simulink model "tp14"  (R2024b)
settings: Solver=ode23t  StartTime=0.0  StopTime=0.2  FixedStep=0.2  RelTol=1e-4  AbsTol=1e-6  EnableMultiTasking=on
undefined symbols (not defined in the file or in its folder): D1, Delta
libraries: spsThreePhaseVIMeasurementLib x28, spsThreePhaseSeriesRLCBranchLib x20, simulink x14, eePMU x14, spsThreePhaseSeriesRLCLoadLib x11, spsThreePhaseSourceLib x5, spsThreePhaseTransformerTwoWindingsLib x5, spspowerguiLib x1
(part 1 of 2)
settings Model: Creator=Bharath  LastModifiedBy=ay988
settings SolverCC: AutoScaleAbsTol=off  MaxConsecutiveMinStep=auto  ZeroCrossControl=DisableAll  AlgebraicLoopSolver=TrustRegion
settings DataIOCC: LimitDataPoints=on  SaveFormat=Array  SignalLoggingSaveFormat=ModelDataLogs  ReturnWorkspaceOutputs=off
settings OptimizationCC: ExpressionDepthLimit=2147483647  LifeSpan=inf
settings DebuggingCC: UnderspecifiedInitializationDetection=Classic  MergeDetectMultiDrivingBlocksExec=none  FcnCallInpInsideContextMsg=warning  UnconnectedInputMsg=warning  UnconnectedOutputMsg=warning  UnconnectedLineMsg=warning  StateNameClashWarn=warning  SFUnexpectedBacktrackingDiag=warning  SFNoUnconditionalDefaultTransitionDiag=warning  SFExecutionAtInitializationDiag=none  ArithmeticOperatorsInVariantConditions=warning
settings HardwareCC: ProdBitPerPointer=32  ProdBitPerSizeT=32  ProdBitPerPtrDiffT=32  ProdLargestAtomicFloat=None  ProdIntDivRoundTo=Undefined  ProdEndianess=Unspecified  ProdWordSize=32  ProdHWDeviceType=32-bit Generic
settings ModelReferenceCC: PropagateSignalLabelsOutOfModel=off
settings SFSimCC: SimUseLocalCustomCode=off  CustomCodeUndefinedFunction=UseInterfaceOnly
settings RTWCC: RTWUseLocalCustomCode=off  GPUComputeCapability=3.5
settings CodeAppCC: StateflowObjectComments=on
settings GRTTargetCC: TargetLangStandard=C89/C90 (ANSI)  CombineOutputUpdateFcns=off  GRTInterface=on
settings ConfigComp: CovMetricSettings=dw  CovSaveCumulativeToWorkspaceVar=on  CovSaveSingleToWorkspaceVar=on  CovExternalEMLEnable=off
settings SimscapeCC: SimscapeNormalizeSystem=off

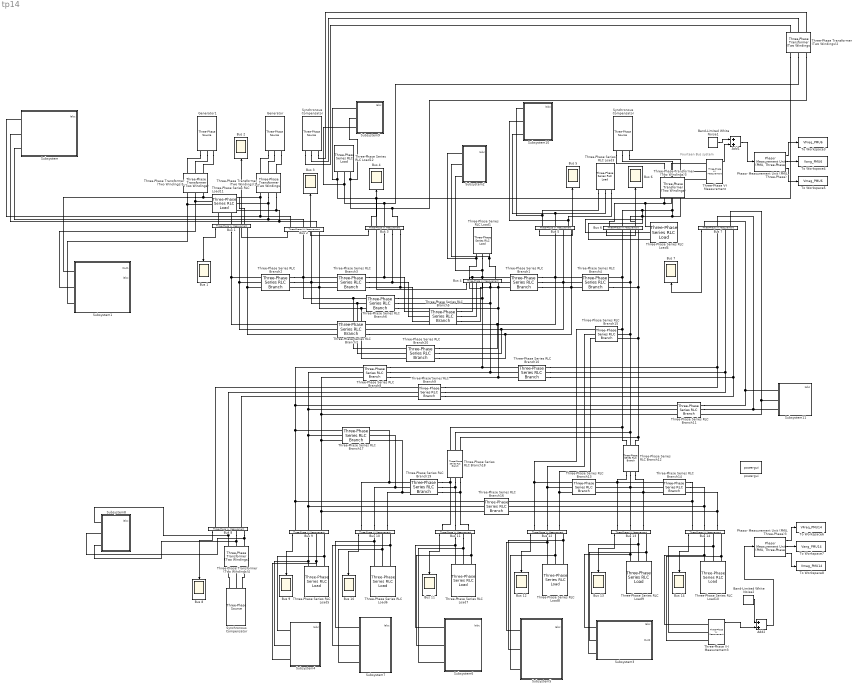
== system tp14 ==
  note: Fourteen Bus system
  " Generator" : spsThreePhaseSourceLib/Three-Phase Source  InternalConnection=Yg  VoltagePhases=off  Voltage=1.045  PhaseAngle=-30  Voltage_phases=[25e3 25e3 25e3]/sqrt(3)  PhaseAngles_phases=[0 -120 +120]  Frequency=50  NonIdealSource=on  SpecifyImpedance=on  Resistance=0.8929  Inductance=16.58e-3  ShortCircuitLevel=10  BaseVoltage=1  XRratio=1  BusType=PV  Pref=0.4  Qref=0  Prefabc=[10e3, 10e3, 10e3]  Qrefabc=[0, 0, 0]  Qmin=-0.4  Qmax=0.5
  " Generator1" : spsThreePhaseSourceLib/Three-Phase Source  InternalConnection=Yg  VoltagePhases=off  Voltage=1.06  PhaseAngle=-30  Voltage_phases=[25e3 25e3 25e3]/sqrt(3)  PhaseAngles_phases=[0 -120 +120]  Frequency=50  NonIdealSource=on  SpecifyImpedance=on  Resistance=0.8929  Inductance=16.58e-3  ShortCircuitLevel=10  BaseVoltage=1  XRratio=1  BusType=PQ  Pref=2.324  Qref=-0.169  Prefabc=[10e3, 10e3, 10e3]  Qrefabc=[0, 0, 0]  Qmin=0  Qmax=0
  Add1 : Sum
  Add2 : Sum
  Band-Limited White Noise1 : simulink/Sources/Band-Limited White Noise  Cov=3.16e-8  Ts=0.00833  seed=[23341]
  Band-Limited White Noise2 : simulink/Sources/Band-Limited White Noise  Cov=3.16e-8  Ts=0.00833  seed=[23341]
  Bus {1..14} (14 alike) : Scope
  "Bus 1 " : spsThreePhaseVIMeasurementLib/Three-Phase V-I Measurement  VoltageMeasurement=phase-to-ground  SetLabelV=off  LabelV=Vabc  Vpu=on  VpuLL=off  CurrentMeasurement=yes  SetLabelI=off  LabelI=Iabc  Ipu=on  Pbase=100e6  Vbase=0.95  OutputType=Complex  PhasorSimulation=off  PSBequivalent=0
  "Bus 10 " : spsThreePhaseVIMeasurementLib/Three-Phase V-I Measurement  VoltageMeasurement=phase-to-ground  SetLabelV=off  LabelV=Vabc  Vpu=on  VpuLL=off  CurrentMeasurement=yes  SetLabelI=off  LabelI=Iabc  Ipu=on  Pbase=100e6  Vbase=0.94  OutputType=Complex  PhasorSimulation=off  PSBequivalent=0
  "Bus 11 " : spsThreePhaseVIMeasurementLib/Three-Phase V-I Measurement  VoltageMeasurement=phase-to-ground  SetLabelV=off  LabelV=Vabc  Vpu=on  VpuLL=off  CurrentMeasurement=yes  SetLabelI=off  LabelI=Iabc  Ipu=on  Pbase=100e6  Vbase=0.95  OutputType=Complex  PhasorSimulation=off  PSBequivalent=0
  "Bus 12 " : spsThreePhaseVIMeasurementLib/Three-Phase V-I Measurement  VoltageMeasurement=phase-to-ground  SetLabelV=off  LabelV=Vabc  Vpu=on  VpuLL=off  CurrentMeasurement=yes  SetLabelI=off  LabelI=Iabc  Ipu=on  Pbase=100e6  Vbase=0.95  OutputType=Complex  PhasorSimulation=off  PSBequivalent=0
  "Bus 13 " : spsThreePhaseVIMeasurementLib/Three-Phase V-I Measurement  VoltageMeasurement=phase-to-ground  SetLabelV=off  LabelV=Vabc  Vpu=on  VpuLL=off  CurrentMeasurement=yes  SetLabelI=off  LabelI=Iabc  Ipu=on  Pbase=100e6  Vbase=0.95  OutputType=Complex  PhasorSimulation=off  PSBequivalent=0
  "Bus 14 " : spsThreePhaseVIMeasurementLib/Three-Phase V-I Measurement  VoltageMeasurement=phase-to-ground  SetLabelV=off  LabelV=Vabc  Vpu=on  VpuLL=off  CurrentMeasurement=yes  SetLabelI=off  LabelI=Iabc  Ipu=on  Pbase=100e6  Vbase=0.92  OutputType=Complex  PhasorSimulation=off  PSBequivalent=0
  "Bus 2 " : spsThreePhaseVIMeasurementLib/Three-Phase V-I Measurement  VoltageMeasurement=phase-to-ground  SetLabelV=off  LabelV=Vabc  Vpu=on  VpuLL=off  CurrentMeasurement=yes  SetLabelI=off  LabelI=Iabc  Ipu=on  Pbase=100e6  Vbase=0.95  OutputType=Complex  PhasorSimulation=off  PSBequivalent=0
  "Bus 3 " : spsThreePhaseVIMeasurementLib/Three-Phase V-I Measurement  VoltageMeasurement=phase-to-ground  SetLabelV=off  LabelV=Vabc  Vpu=on  VpuLL=off  CurrentMeasurement=yes  SetLabelI=off  LabelI=Iabc  Ipu=on  Pbase=100e6  Vbase=0.95  OutputType=Complex  PhasorSimulation=off  PSBequivalent=0
  "Bus 4 " : spsThreePhaseVIMeasurementLib/Three-Phase V-I Measurement  VoltageMeasurement=phase-to-ground  SetLabelV=off  LabelV=Vabc  Vpu=on  VpuLL=off  CurrentMeasurement=yes  SetLabelI=off  LabelI=Iabc  Ipu=on  Pbase=100e6  Vbase=0.95  OutputType=Complex  PhasorSimulation=off  PSBequivalent=0
  "Bus 5 " : spsThreePhaseVIMeasurementLib/Three-Phase V-I Measurement  VoltageMeasurement=phase-to-ground  SetLabelV=off  LabelV=Vabc  Vpu=on  VpuLL=off  CurrentMeasurement=yes  SetLabelI=off  LabelI=Iabc  Ipu=on  Pbase=100e6  Vbase=0.95  OutputType=Complex  PhasorSimulation=off  PSBequivalent=0
  "Bus 6 " : spsThreePhaseVIMeasurementLib/Three-Phase V-I Measurement  VoltageMeasurement=phase-to-ground  SetLabelV=off  LabelV=Vabc  Vpu=on  VpuLL=off  CurrentMeasurement=yes  SetLabelI=off  LabelI=Iabc  Ipu=on  Pbase=100e6  Vbase=0.95  OutputType=Complex  PhasorSimulation=off  PSBequivalent=0
  "Bus 7 " : spsThreePhaseVIMeasurementLib/Three-Phase V-I Measurement  VoltageMeasurement=phase-to-ground  SetLabelV=off  LabelV=Vabc  Vpu=on  VpuLL=off  CurrentMeasurement=yes  SetLabelI=off  LabelI=Iabc  Ipu=off  Pbase=100e6  Vbase=0.95  OutputType=Complex  PhasorSimulation=off  PSBequivalent=0
  "Bus 8 " : spsThreePhaseVIMeasurementLib/Three-Phase V-I Measurement  VoltageMeasurement=phase-to-ground  SetLabelV=off  LabelV=Vabc  Vpu=on  VpuLL=off  CurrentMeasurement=yes  SetLabelI=off  LabelI=Iabc  Ipu=on  Pbase=100e6  Vbase=1  OutputType=Complex  PhasorSimulation=off  PSBequivalent=0
  "Bus 9 " : spsThreePhaseVIMeasurementLib/Three-Phase V-I Measurement  VoltageMeasurement=phase-to-ground  SetLabelV=off  LabelV=Vabc  Vpu=on  VpuLL=off  CurrentMeasurement=yes  SetLabelI=off  LabelI=Iabc  Ipu=on  Pbase=100e6  Vbase=0.94  OutputType=Complex  PhasorSimulation=off  PSBequivalent=0
  "Phasor Measurement Unit (PMU, Three-Phase)" : eePMU/Phasor Measurement Unit (PMU, Three-Phase)  frequency=60  Nsr=64  k=2
      settings: LibrarySourceBlock=|
      | ee_sl_lib/Measurements/Phasor Measurement Unit
      | (PMU, Three-Phase)
  "Phasor Measurement Unit (PMU, Three-Phase)3" : eePMU/Phasor Measurement Unit (PMU, Three-Phase)  frequency=60  Nsr=64  k=2
      settings: LibrarySourceBlock=|
      | ee_sl_lib/Measurements/Phasor Measurement Unit
      | (PMU, Three-Phase)
  Subsystem : Subsystem
  Subsystem1 : Subsystem
  Subsystem10 : Subsystem
  Subsystem11 : Subsystem
  Subsystem2 : Subsystem
  Subsystem3 : Subsystem
      settings: PortSchema="{\"entries\":[{\"content\":{\"sides\":[{\"content\":{\"connectorIds\":[\"LConn1\",\"LConn2\",\"LConn3\"]},\"type\":\"ConnectorPlacement.EquallySpacedRectSide\",\"uuid\":\"0f5ea291-c895-42b3-b291-256dbc806b24\"},{\"content\":{\"connectorIds\":[\"Out1\",\"RConn1\",\"Out2\",\"RConn2\",\"RConn3\"],\"side\":\"RIGHT\"},\"type\":\"ConnectorPlacement.EquallySpacedRectSide\",\"uuid\":\"58815e83-7991-43ed-9f07-61d24ff721cc\"},{\"content\":{\"side\":\"TOP\"},\"type\":\"ConnectorPlacement.EquallySpacedRectSide\",\"uuid\":\"ed2c6d76-d5b4-4f96-9a90-a27dace25e5a\"}]},\"type\":\"ConnectorPlacement.EquallySpacedConnector\",\"uuid\":\"17b272e0-abde-4b35-9582-c71450a7a318\"}],\"packageUris\":[\"http://schema.mathworks.com/mf0/Connector/R2020b\"],\"version\":\"1.0\"}"
  Subsystem4 : Subsystem
  Subsystem5 : Subsystem
  Subsystem6 : Subsystem
  Subsystem7 : Subsystem
  Subsystem8 : Subsystem
  Subsystem9 : Subsystem
  Synchronous Compensator : spsThreePhaseSourceLib/Three-Phase Source  InternalConnection=Yg  VoltagePhases=off  Voltage=1.09  PhaseAngle=-30  Voltage_phases=[25e3 25e3 25e3]/sqrt(3)  PhaseAngles_phases=[0 -120 +120]  Frequency=50  NonIdealSource=on  SpecifyImpedance=on  Resistance=0.8929  Inductance=16.58e-3  ShortCircuitLevel=10  BaseVoltage=1  XRratio=1  BusType=PV  Pref=0  Qref=0  Prefabc=[10e3, 10e3, 10e3]  Qrefabc=[0, 0, 0]  Qmin=-0.06  Qmax=0.24
  Synchronous Compensator : spsThreePhaseSourceLib/Three-Phase Source  InternalConnection=Yg  VoltagePhases=off  Voltage=1.01  PhaseAngle=-30  Voltage_phases=[25e3 25e3 25e3]/sqrt(3)  PhaseAngles_phases=[0 -120 +120]  Frequency=50  NonIdealSource=on  SpecifyImpedance=on  Resistance=0.8929  Inductance=16.58e-3  ShortCircuitLevel=10  BaseVoltage=1  XRratio=1  BusType=PV  Pref=0  Qref=23.4e6  Prefabc=[10e3, 10e3, 10e3]  Qrefabc=[0, 0, 0]  Qmin=0  Qmax=0.4
  "Synchronous Compensator " : spsThreePhaseSourceLib/Three-Phase Source  InternalConnection=Yg  VoltagePhases=off  Voltage=1.07  PhaseAngle=-30  Voltage_phases=[25e3 25e3 25e3]/sqrt(3)  PhaseAngles_phases=[0 -120 +120]  Frequency=50  NonIdealSource=on  SpecifyImpedance=on  Resistance=0.8929  Inductance=16.58e-3  ShortCircuitLevel=10  BaseVoltage=1  XRratio=1  BusType=PV  Pref=0  Qref=23.4e6  Prefabc=[10e3, 10e3, 10e3]  Qrefabc=[0, 0, 0]  Qmin=-0.06  Qmax=0.24
  Three-Phase Series RLC Branch1 : spsThreePhaseSeriesRLCBranchLib/Three-Phase Series RLC Branch  LConnTagsString=A|B|C  RConnTagsString=A|B|C  BranchType=RLC  Resistance=0.01335  Inductance=0.04211/(2*pi*50)  Capacitance=1/0.0128/(2*pi*50)  Measurements=None
  Three-Phase Series RLC Branch10 : spsThreePhaseSeriesRLCBranchLib/Three-Phase Series RLC Branch  LConnTagsString=A|B|C  RConnTagsString=A|B|C  BranchType=L  Resistance=1  Inductance=0.20912/(2*pi*50)  Capacitance=1e-6  Measurements=None
  Three-Phase Series RLC Branch11 : spsThreePhaseSeriesRLCBranchLib/Three-Phase Series RLC Branch  LConnTagsString=A|B|C  RConnTagsString=A|B|C  BranchType=L  Resistance=1  Inductance=0.11001/(2*pi*50)  Capacitance=1e-6  Measurements=None
  Three-Phase Series RLC Branch12 : spsThreePhaseSeriesRLCBranchLib/Three-Phase Series RLC Branch  LConnTagsString=A|B|C  RConnTagsString=A|B|C  BranchType=RL  Resistance=0.06615  Inductance=0.13027/(2*pi*50)  Capacitance=1e-6  Measurements=None
  Three-Phase Series RLC Branch13 : spsThreePhaseSeriesRLCBranchLib/Three-Phase Series RLC Branch  LConnTagsString=A|B|C  RConnTagsString=A|B|C  BranchType=RL  Resistance=0.22092  Inductance=0.19988/(2*pi*50)  Capacitance=1e-6  Measurements=None
  Three-Phase Series RLC Branch14 : spsThreePhaseSeriesRLCBranchLib/Three-Phase Series RLC Branch  LConnTagsString=A|B|C  RConnTagsString=A|B|C  BranchType=RL  Resistance=0.17093  Inductance=0.34802/(2*pi*50)  Capacitance=1e-6  Measurements=None
  Three-Phase Series RLC Branch15 : spsThreePhaseSeriesRLCBranchLib/Three-Phase Series RLC Branch  LConnTagsString=A|B|C  RConnTagsString=A|B|C  BranchType=RL  Resistance=0.12291  Inductance=0.25581/(2*pi*50)  Capacitance=1e-6  Measurements=None
  Three-Phase Series RLC Branch16 : spsThreePhaseSeriesRLCBranchLib/Three-Phase Series RLC Branch  LConnTagsString=A|B|C  RConnTagsString=A|B|C  BranchType=RL  Resistance=0.12711  Inductance=0.27038/(2*pi*50)  Capacitance=1e-6  Measurements=None
  Three-Phase Series RLC Branch17 : spsThreePhaseSeriesRLCBranchLib/Three-Phase Series RLC Branch  LConnTagsString=A|B|C  RConnTagsString=A|B|C  BranchType=RL  Resistance=0.03181  Inductance=0.08450/(2*pi*50)  Capacitance=1e-6  Measurements=None
  Three-Phase Series RLC Branch18 : spsThreePhaseSeriesRLCBranchLib/Three-Phase Series RLC Branch  LConnTagsString=A|B|C  RConnTagsString=A|B|C  BranchType=RL  Resistance=0.09498  Inductance=0.1989/(2*pi*50)  Capacitance=1e-6  Measurements=None
  Three-Phase Series RLC Branch19 : spsThreePhaseSeriesRLCBranchLib/Three-Phase Series RLC Branch  LConnTagsString=A|B|C  RConnTagsString=A|B|C  BranchType=RL  Resistance=0.08205  Inductance=0.19207/(2*pi*50)  Capacitance=1e-6  Measurements=None
  Three-Phase Series RLC Branch2 : spsThreePhaseSeriesRLCBranchLib/Three-Phase Series RLC Branch  LConnTagsString=A|B|C  RConnTagsString=A|B|C  BranchType=RLC  Resistance=0.01938  Inductance=0.05917/(2*pi*50)  Capacitance=1/0.0528/(2*pi*50)  Measurements=None
  Three-Phase Series RLC Branch20 : spsThreePhaseSeriesRLCBranchLib/Three-Phase Series RLC Branch  LConnTagsString=A|B|C  RConnTagsString=A|B|C  BranchType=RLC  Resistance=0.05695  Inductance=0.17388/(2*pi*50)  Capacitance=1/0.0340/(2*pi*50)  Measurements=None
  Three-Phase Series RLC Branch3 : spsThreePhaseSeriesRLCBranchLib/Three-Phase Series RLC Branch  LConnTagsString=A|B|C  RConnTagsString=A|B|C  BranchType=RLC  Resistance=0.04699  Inductance=0.19797/(2*pi*50)  Capacitance=1/0.0438/(2*pi*50)  Measurements=None
  Three-Phase Series RLC Branch4 : spsThreePhaseSeriesRLCBranchLib/Three-Phase Series RLC Branch  LConnTagsString=A|B|C  RConnTagsString=A|B|C  BranchType=L  Resistance=1  Inductance=0.25202/(2*pi*50)  Capacitance=1e-6  Measurements=None
  Three-Phase Series RLC Branch5 : spsThreePhaseSeriesRLCBranchLib/Three-Phase Series RLC Branch  LConnTagsString=A|B|C  RConnTagsString=A|B|C  BranchType=RLC  Resistance=0.06701  Inductance=0.17103/(2*pi*50)  Capacitance=1/0.0346/(2*pi*50)  Measurements=None
  Three-Phase Series RLC Branch6 : spsThreePhaseSeriesRLCBranchLib/Three-Phase Series RLC Branch  LConnTagsString=A|B|C  RConnTagsString=A|B|C  BranchType=RLC  Resistance=0.05811  Inductance=0.17632/(2*pi*50)  Capacitance=1/0.0374/(2*pi*50)  Measurements=None
  Three-Phase Series RLC Branch7 : spsThreePhaseSeriesRLCBranchLib/Three-Phase Series RLC Branch  LConnTagsString=A|B|C  RConnTagsString=A|B|C  BranchType=RLC  Resistance=0.05403  Inductance=0.22304/(2*pi*50)  Capacitance=1/0.0492/(2*pi*50)  Measurements=None
  Three-Phase Series RLC Branch8 : spsThreePhaseSeriesRLCBranchLib/Three-Phase Series RLC Branch  LConnTagsString=A|B|C  RConnTagsString=A|B|C  BranchType=L  Resistance=1  Inductance=0.55618/(2*pi*50)  Capacitance=1e-6  Measurements=None
  Three-Phase Series RLC Branch9 : spsThreePhaseSeriesRLCBranchLib/Three-Phase Series RLC Branch  LConnTagsString=A|B|C  RConnTagsString=A|B|C  BranchType=L  Resistance=1  Inductance=0.17615/(2*pi*50)  Capacitance=1e-6  Measurements=None
  Three-Phase Series RLC Load1 : spsThreePhaseSeriesRLCLoadLib/Three-Phase Series RLC Load  LConnTagsString=A|B|C  Configuration=Y (grounded)  NominalVoltage=1  Vabc=[1e3 1e3 1e3]  Vabcp=[1e3 1e3 1e3]  NominalFrequency=50  UnbalancedPower=off  ActivePower=0.478  InductivePower=0  CapacitivePower=0.039  Pabc=[10e3 9e3 11e3]  QLabc=[100 90 110]  QCabc=[100 90 110]  Pabcp=[10e3 9e3 11e3]  QLabcp=[100 90 110]  QCabcp=[100 90 110]  Measurements=None  LoadType=constant PQ
  Three-Phase Series RLC Load10 : spsThreePhaseSeriesRLCLoadLib/Three-Phase Series RLC Load  LConnTagsString=A|B|C  Configuration=Y (grounded)  NominalVoltage=1  Vabc=[1e3 1e3 1e3]  Vabcp=[1e3 1e3 1e3]  NominalFrequency=50  UnbalancedPower=off  ActivePower=0.149  InductivePower=0.050  CapacitivePower=0  Pabc=[10e3 9e3 11e3]  QLabc=[100 90 110]  QCabc=[100 90 110]  Pabcp=[10e3 9e3 11e3]  QLabcp=[100 90 110]  QCabcp=[100 90 110]  Measurements=None  LoadType=constant Z
  Three-Phase Series RLC Load11 : spsThreePhaseSeriesRLCLoadLib/Three-Phase Series RLC Load  LConnTagsString=A|B|C  Configuration=Y (grounded)  NominalVoltage=1  Vabc=[1e3 1e3 1e3]  Vabcp=[1e3 1e3 1e3]  NominalFrequency=50  UnbalancedPower=off  ActivePower=0.217  InductivePower=0.127  CapacitivePower=0  Pabc=[10e3 9e3 11e3]  QLabc=[100 90 110]  QCabc=[100 90 110]  Pabcp=[10e3 9e3 11e3]  QLabcp=[100 90 110]  QCabcp=[100 90 110]  Measurements=None  LoadType=constant PQ
  Three-Phase Series RLC Load12 : spsThreePhaseSeriesRLCLoadLib/Three-Phase Series RLC Load  LConnTagsString=A|B|C  Configuration=Y (grounded)  NominalVoltage=1  Vabc=[1e3 1e3 1e3]  Vabcp=[1e3 1e3 1e3]  NominalFrequency=50  UnbalancedPower=off  ActivePower=0.942  InductivePower=0.191  CapacitivePower=0  Pabc=[10e3 9e3 11e3]  QLabc=[100 90 110]  QCabc=[100 90 110]  Pabcp=[10e3 9e3 11e3]  QLabcp=[100 90 110]  QCabcp=[100 90 110]  Measurements=None  LoadType=constant PQ
  Three-Phase Series RLC Load3 : spsThreePhaseSeriesRLCLoadLib/Three-Phase Series RLC Load  LConnTagsString=A|B|C  Configuration=Y (grounded)  NominalVoltage=1  Vabc=[1e3 1e3 1e3]  Vabcp=[1e3 1e3 1e3]  NominalFrequency=50  UnbalancedPower=off  ActivePower=0.076  InductivePower=0.016  CapacitivePower=0  Pabc=[10e3 9e3 11e3]  QLabc=[100 90 110]  QCabc=[100 90 110]  Pabcp=[10e3 9e3 11e3]  QLabcp=[100 90 110]  QCabcp=[100 90 110]  Measurements=None  LoadType=constant PQ
  Three-Phase Series RLC Load4 : spsThreePhaseSeriesRLCLoadLib/Three-Phase Series RLC Load  LConnTagsString=A|B|C  Configuration=Y (grounded)  NominalVoltage=1  Vabc=[1e3 1e3 1e3]  Vabcp=[1e3 1e3 1e3]  NominalFrequency=50  UnbalancedPower=off  ActivePower=0.112  InductivePower=0.075  CapacitivePower=0  Pabc=[10e3 9e3 11e3]  QLabc=[100 90 110]  QCabc=[100 90 110]  Pabcp=[10e3 9e3 11e3]  QLabcp=[100 90 110]  QCabcp=[100 90 110]  Measurements=None  LoadType=constant PQ
  Three-Phase Series RLC Load5 : spsThreePhaseSeriesRLCLoadLib/Three-Phase Series RLC Load  LConnTagsString=A|B|C  Configuration=Y (grounded)  NominalVoltage=1  Vabc=[1e3 1e3 1e3]  Vabcp=[1e3 1e3 1e3]  NominalFrequency=50  UnbalancedPower=off  ActivePower=0.295  InductivePower=0.166  CapacitivePower=0  Pabc=[10e3 9e3 11e3]  QLabc=[100 90 110]  QCabc=[100 90 110]  Pabcp=[10e3 9e3 11e3]  QLabcp=[100 90 110]  QCabcp=[100 90 110]  Measurements=None  LoadType=constant PQ
  Three-Phase Series RLC Load6 : spsThreePhaseSeriesRLCLoadLib/Three-Phase Series RLC Load  LConnTagsString=A|B|C  Configuration=Y (grounded)  NominalVoltage=1  Vabc=[1e3 1e3 1e3]  Vabcp=[1e3 1e3 1e3]  NominalFrequency=50  UnbalancedPower=off  ActivePower=0.09  InductivePower=0.058  CapacitivePower=0  Pabc=[10e3 9e3 11e3]  QLabc=[100 90 110]  QCabc=[100 90 110]  Pabcp=[10e3 9e3 11e3]  QLabcp=[100 90 110]  QCabcp=[100 90 110]  Measurements=None  LoadType=constant PQ
  Three-Phase Series RLC Load7 : spsThreePhaseSeriesRLCLoadLib/Three-Phase Series RLC Load  LConnTagsString=A|B|C  Configuration=Y (grounded)  NominalVoltage=1  Vabc=[1e3 1e3 1e3]  Vabcp=[1e3 1e3 1e3]  NominalFrequency=50  UnbalancedPower=off  ActivePower=0.035  InductivePower=0.018  CapacitivePower=0  Pabc=[10e3 9e3 11e3]  QLabc=[100 90 110]  QCabc=[100 90 110]  Pabcp=[10e3 9e3 11e3]  QLabcp=[100 90 110]  QCabcp=[100 90 110]  Measurements=None  LoadType=constant PQ
  Three-Phase Series RLC Load8 : spsThreePhaseSeriesRLCLoadLib/Three-Phase Series RLC Load  LConnTagsString=A|B|C  Configuration=Y (grounded)  NominalVoltage=1  Vabc=[1e3 1e3 1e3]  Vabcp=[1e3 1e3 1e3]  NominalFrequency=50  UnbalancedPower=off  ActivePower=0.061  InductivePower=0.016  CapacitivePower=0  Pabc=[10e3 9e3 11e3]  QLabc=[100 90 110]  QCabc=[100 90 110]  Pabcp=[10e3 9e3 11e3]  QLabcp=[100 90 110]  QCabcp=[100 90 110]  Measurements=None  LoadType=constant PQ
  Three-Phase Series RLC Load9 : spsThreePhaseSeriesRLCLoadLib/Three-Phase Series RLC Load  LConnTagsString=A|B|C  Configuration=Y (grounded)  NominalVoltage=1  Vabc=[1e3 1e3 1e3]  Vabcp=[1e3 1e3 1e3]  NominalFrequency=50  UnbalancedPower=off  ActivePower=0.135  InductivePower=0.058  CapacitivePower=0  Pabc=[10e3 9e3 11e3]  QLabc=[100 90 110]  QCabc=[100 90 110]  Pabcp=[10e3 9e3 11e3]  QLabcp=[100 90 110]  QCabcp=[100 90 110]  Measurements=None  LoadType=constant PQ
  Three-Phase Transformer (Two Windings)1 : spsThreePhaseTransformerTwoWindingsLib/Three-Phase Transformer (Two Windings)  Winding1Connection=Delta (D1)  Winding2Connection=Yg  CoreType=Three single-phase transformers  SetSaturation=off  Hysteresis=off  DataFile='hysteresis'  SetInitialFlux=off  Measurements=None  UNITS=pu  NominalPower=[ 1 , 50 ]  Winding1=[ 1.045 , 0.002 , 0.08 ]  Winding2=[ 1.045 , 0.002 , 0.08 ]  Rm=500  Lm=500  L0=0.5  Saturation=[ 0,0 ; 0.0024,1.2 ; 1.0,1.52 ]  InitialFluxes=[ 0.8 , -0.8 , 0.7 ]  BreakLoop=off  DiscreteSolver=Trapezoidal iterative  DataType=off  TransfoNumber=1
  Three-Phase Transformer (Two Windings)2 : spsThreePhaseTransformerTwoWindingsLib/Three-Phase Transformer (Two Windings)  Winding1Connection=Delta (D1)  Winding2Connection=Yg  CoreType=Three single-phase transformers  SetSaturation=off  Hysteresis=off  DataFile='hysteresis'  SetInitialFlux=off  Measurements=None  UNITS=pu  NominalPower=[ 1 , 50 ]  Winding1=[ 1.01 , 0.002 , 0.08 ]  Winding2=[ 1.01 , 0.002 , 0.08 ]  Rm=500  Lm=500  L0=0.5  Saturation=[ 0,0 ; 0.0024,1.2 ; 1.0,1.52 ]  InitialFluxes=[ 0.8 , -0.8 , 0.7 ]  BreakLoop=off  DiscreteSolver=Trapezoidal iterative  DataType=off  TransfoNumber=1
  Three-Phase Transformer (Two Windings)3 : spsThreePhaseTransformerTwoWindingsLib/Three-Phase Transformer (Two Windings)  Winding1Connection=Delta (D1)  Winding2Connection=Yg  CoreType=Three single-phase transformers  SetSaturation=off  Hysteresis=off  DataFile='hysteresis'  SetInitialFlux=off  Measurements=None  UNITS=pu  NominalPower=[ 1 , 50 ]  Winding1=[ 1.07 , 0.002 , 0.08 ]  Winding2=[ 1.07 , 0.002 , 0.08 ]  Rm=500  Lm=500  L0=0.5  Saturation=[ 0,0 ; 0.0024,1.2 ; 1.0,1.52 ]  InitialFluxes=[ 0.8 , -0.8 , 0.7 ]  BreakLoop=off  DiscreteSolver=Trapezoidal iterative  DataType=off  TransfoNumber=1
  Three-Phase Transformer (Two Windings)4 : spsThreePhaseTransformerTwoWindingsLib/Three-Phase Transformer (Two Windings)  Winding1Connection=Yg  Winding2Connection=Delta (D1)  CoreType=Three single-phase transformers  SetSaturation=off  Hysteresis=off  DataFile='hysteresis'  SetInitialFlux=off  Measurements=None  UNITS=pu  NominalPower=[ 1 , 50 ]  Winding1=[ 1.09 , 0.002 , 0.08]  Winding2=[1.09 , 0.002 , 0.08]  Rm=500  Lm=500  L0=0.5  Saturation=[0 0;0.0023999 1.2;1 1.52]  InitialFluxes=[0.80002 -0.80002 0.69999]  BreakLoop=off  DiscreteSolver=Trapezoidal iterative  DataType=off  TransfoNumber=1
  Three-Phase Transformer (Two Windings)5 : spsThreePhaseTransformerTwoWindingsLib/Three-Phase Transformer (Two Windings)  Winding1Connection=Delta (D1)  Winding2Connection=Yg  CoreType=Three single-phase transformers  SetSaturation=off  Hysteresis=off  DataFile='hysteresis'  SetInitialFlux=off  Measurements=None  UNITS=pu  NominalPower=[ 1 , 50 ]  Winding1=[ 1.06 , 0.002 , 0.08 ]  Winding2=[ 1.06 , 0.002 , 0.08 ]  Rm=500  Lm=500  L0=0.5  Saturation=[ 0,0 ; 0.0024,1.2 ; 1.0,1.52 ]  InitialFluxes=[ 0.8 , -0.8 , 0.7 ]  BreakLoop=off  DiscreteSolver=Trapezoidal iterative  DataType=off  TransfoNumber=1
  Three-Phase V-I Measurement : spsThreePhaseVIMeasurementLib/Three-Phase V-I Measurement  VoltageMeasurement=phase-to-ground  SetLabelV=off  LabelV=Vabc  Vpu=off  VpuLL=off  CurrentMeasurement=yes  SetLabelI=off  LabelI=Iabc  Ipu=off  Pbase=100e6  Vbase=500e3  OutputType=Complex  PhasorSimulation=off  PSBequivalent=0
  Three-Phase V-I Measurement3 : spsThreePhaseVIMeasurementLib/Three-Phase V-I Measurement  VoltageMeasurement=phase-to-ground  SetLabelV=off  LabelV=Vabc  Vpu=off  VpuLL=off  CurrentMeasurement=yes  SetLabelI=off  LabelI=Iabc  Ipu=off  Pbase=100e6  Vbase=500e3  OutputType=Complex  PhasorSimulation=off  PSBequivalent=0
  To Workspace3 : ToWorkspace  VariableName=VFreq_PMU6  SaveFormat=Timeseries  SampleTime=-1
  To Workspace4 : ToWorkspace  VariableName=Vang_PMU6  SaveFormat=Timeseries  SampleTime=-1
  To Workspace5 : ToWorkspace  VariableName=Vmag_PMU6  SaveFormat=Timeseries  SampleTime=-1
  To Workspace6 : ToWorkspace  VariableName=VFreq_PMU14  SaveFormat=Timeseries  SampleTime=-1
  To Workspace7 : ToWorkspace  VariableName=Vang_PMU14  SaveFormat=Timeseries  SampleTime=-1
  To Workspace8 : ToWorkspace  VariableName=Vmag_PMU14  SaveFormat=Timeseries  SampleTime=-1
  powergui : spspowerguiLib/powergui  Priority=1  SimulationMode=Continuous  SampleTime=50e-6  frequency=60  Iterations=50  frequencyindice=50  Pbase=100e6  ErrMax=1e-4  UnitsV=kV  UnitsW=MW  buscounter=0  FunctionMessages=off  echomessages=off  EnableUseOfTLC=off  CurrentSourceSwitches=on  DisableSnubberDevices=off  DisableRonSwitches=off  DisableVfSwitches=off  DisplayEquations=off  AutomaticDiscreteSolvers=off  SolverType=Tustin  Interpol=off  ExternalGateDelay=off  methode=off  Ts=100  x0status=blocks  SPID=off  SwTol=0  HookPort=off  NonlinearTolerance=1e-4  nMaxIteration=100  ContinueOnMaxIteration=off  RestoreLinks=warning  ResistiveCurrentMeasurement=off  Frange=[0:2:500]  Ylog=off  Xlog=on  ShowGrid=off  save=off  variable=ZData  structure=0  ZoomFFT=off  StartTime=0.0  cycles=1  DisplayStyle=1  fundamental=60  FreqAxis=off  MaxFrequency=1000  frequencyindicesteady=1  RmsSteady=1  display=off
  wires:
  "Bus 11 "/1 -> Bus 11/1
  "Bus 10 "/1 -> Bus 10/1
  "Bus 9 "/1 -> Bus 9/1
  "Bus 8 "/1 -> Bus 8/1
  "Bus 7 "/1 -> Bus 7/1
  "Bus 4 "/1 -> Bus 4/1
  "Bus 2 "/1 -> Bus 2/1
  "Bus 14 "/1 -> Bus 14/1
  "Bus 13 "/1 -> Bus 13/1
  "Bus 12 "/1 -> Bus 12/1
  "Bus 5 "/1 -> Bus 5/1
  "Bus 1 "/1 -> Bus 1/1
  "Bus 3 "/1 -> Bus 3/1
  "Bus 6 "/1 -> Bus 6/1
  Band-Limited White Noise1/1 -> Add1/1
  Three-Phase V-I Measurement/1 -> Add1/2
  Add1/1 -> "Phasor Measurement Unit (PMU, Three-Phase)"/1
  Three-Phase V-I Measurement3/1 -> Add2/2
  Band-Limited White Noise2/1 -> Add2/1
  Add2/1 -> "Phasor Measurement Unit (PMU, Three-Phase)3"/1
  "Phasor Measurement Unit (PMU, Three-Phase)"/1 -> To Workspace3/1
  "Phasor Measurement Unit (PMU, Three-Phase)"/2 -> To Workspace4/1
  "Phasor Measurement Unit (PMU, Three-Phase)"/3 -> To Workspace5/1
  "Phasor Measurement Unit (PMU, Three-Phase)3"/1 -> To Workspace6/1
  "Phasor Measurement Unit (PMU, Three-Phase)3"/2 -> To Workspace7/1
  "Phasor Measurement Unit (PMU, Three-Phase)3"/3 -> To Workspace8/1
  connections:
  "Bus 9 "/LConn3 -- Three-Phase Series RLC Branch16/RConn3 -- Three-Phase Series RLC Branch17/RConn3 -- Three-Phase Series RLC Branch11/RConn3 -- Three-Phase Series RLC Branch8/LConn3
  "Bus 9 "/LConn2 -- Three-Phase Series RLC Branch16/RConn2 -- Three-Phase Series RLC Branch17/RConn2 -- Three-Phase Series RLC Branch11/RConn2 -- Three-Phase Series RLC Branch8/LConn2
  "Bus 9 "/LConn1 -- Three-Phase Series RLC Branch16/RConn1 -- Three-Phase Series RLC Branch17/RConn1 -- Three-Phase Series RLC Branch11/RConn1 -- Three-Phase Series RLC Branch8/LConn1
  "Bus 7 "/RConn3 -- Three-Phase Series RLC Branch10/RConn3 -- Three-Phase Series RLC Branch9/RConn3
  "Bus 7 "/RConn2 -- Three-Phase Series RLC Branch10/RConn2 -- Three-Phase Series RLC Branch9/RConn2
  "Bus 7 "/RConn1 -- Three-Phase Series RLC Branch10/RConn1 -- Three-Phase Series RLC Branch9/RConn1
  "Bus 6 "/RConn3 -- Three-Phase Series RLC Branch4/RConn3 -- Three-Phase Series RLC Branch12/LConn3 -- Three-Phase Series RLC Branch18/LConn3 -- Three-Phase Series RLC Branch15/LConn3
  "Bus 6 "/RConn2 -- Three-Phase Series RLC Branch15/LConn2 -- Three-Phase Series RLC Branch18/LConn2 -- Three-Phase Series RLC Branch12/LConn2 -- Three-Phase Series RLC Branch4/RConn2
  "Bus 6 "/RConn1 -- Three-Phase Series RLC Branch12/LConn1 -- Three-Phase Series RLC Branch18/LConn1 -- Three-Phase Series RLC Branch15/LConn1 -- Three-Phase Series RLC Branch4/RConn1
  "Bus 5 "/RConn3 -- Three-Phase Series RLC Branch20/RConn3 -- Three-Phase Series RLC Branch7/RConn3 -- Three-Phase Series RLC Branch1/RConn3 -- Three-Phase Series RLC Branch4/LConn3
  "Bus 5 "/RConn2 -- Three-Phase Series RLC Branch20/RConn2 -- Three-Phase Series RLC Branch7/RConn2 -- Three-Phase Series RLC Branch1/RConn2 -- Three-Phase Series RLC Branch4/LConn2
  "Bus 5 "/RConn1 -- Three-Phase Series RLC Branch20/RConn1 -- Three-Phase Series RLC Branch7/RConn1 -- Three-Phase Series RLC Branch1/RConn1 -- Three-Phase Series RLC Branch4/LConn1
  "Bus 3 "/RConn2 -- Three-Phase Series RLC Branch5/LConn2 -- Three-Phase Series RLC Branch3/RConn2
  "Bus 3 "/RConn1 -- Three-Phase Series RLC Branch5/LConn1 -- Three-Phase Series RLC Branch3/RConn1
  "Bus 2 "/RConn3 -- Three-Phase Series RLC Branch20/LConn3 -- Three-Phase Series RLC Branch6/LConn3 -- Three-Phase Series RLC Branch3/LConn3 -- Three-Phase Series RLC Branch2/RConn3
  "Bus 2 "/RConn2 -- Three-Phase Series RLC Branch20/LConn2 -- Three-Phase Series RLC Branch6/LConn2 -- Three-Phase Series RLC Branch2/RConn2 -- Three-Phase Series RLC Branch3/LConn2
  "Bus 2 "/RConn1 -- Three-Phase Series RLC Branch20/LConn1 -- Three-Phase Series RLC Branch6/LConn1 -- Three-Phase Series RLC Branch2/RConn1 -- Three-Phase Series RLC Branch3/LConn1
  Three-Phase Series RLC Load11/LConn1 -- Three-Phase Transformer (Two Windings)1/RConn1 -- "Bus 2 "/LConn1 -- Subsystem/LConn1
  "Bus 14 "/LConn3 -- Three-Phase Series RLC Branch16/LConn3 -- Three-Phase Series RLC Branch14/LConn3
  "Bus 14 "/LConn2 -- Three-Phase Series RLC Branch16/LConn2 -- Three-Phase Series RLC Branch14/LConn2
  "Bus 14 "/LConn1 -- Three-Phase Series RLC Branch16/LConn1 -- Three-Phase Series RLC Branch14/LConn1
  "Bus 13 "/LConn3 -- Three-Phase Series RLC Branch14/RConn3 -- Three-Phase Series RLC Branch13/LConn3 -- Three-Phase Series RLC Branch12/RConn3
  "Bus 13 "/LConn2 -- Three-Phase Series RLC Branch14/RConn2 -- Three-Phase Series RLC Branch12/RConn2 -- Three-Phase Series RLC Branch13/LConn2
  "Bus 13 "/LConn1 -- Three-Phase Series RLC Branch14/RConn1 -- Three-Phase Series RLC Branch12/RConn1 -- Three-Phase Series RLC Branch13/LConn1
  "Bus 12 "/LConn3 -- Three-Phase Series RLC Branch13/RConn3 -- Three-Phase Series RLC Branch15/RConn3
  "Bus 12 "/LConn2 -- Three-Phase Series RLC Branch13/RConn2 -- Three-Phase Series RLC Branch15/RConn2
  "Bus 12 "/LConn1 -- Three-Phase Series RLC Branch13/RConn1 -- Three-Phase Series RLC Branch15/RConn1
  "Bus 11 "/LConn3 -- Three-Phase Series RLC Branch19/RConn3 -- Three-Phase Series RLC Branch18/RConn3
  "Bus 11 "/LConn2 -- Three-Phase Series RLC Branch19/RConn2 -- Three-Phase Series RLC Branch18/RConn2
  "Bus 11 "/LConn1 -- Three-Phase Series RLC Branch19/RConn1 -- Three-Phase Series RLC Branch18/RConn1
  "Bus 10 "/LConn3 -- Three-Phase Series RLC Branch17/LConn3 -- Three-Phase Series RLC Branch19/LConn3
  "Bus 10 "/LConn2 -- Three-Phase Series RLC Branch17/LConn2 -- Three-Phase Series RLC Branch19/LConn2
  "Bus 10 "/LConn1 -- Three-Phase Series RLC Branch17/LConn1 -- Three-Phase Series RLC Branch19/LConn1
  "Bus 1 "/RConn3 -- Three-Phase Series RLC Branch2/LConn3 -- Three-Phase Series RLC Branch7/LConn3
  "Bus 1 "/RConn2 -- Three-Phase Series RLC Branch2/LConn2 -- Three-Phase Series RLC Branch7/LConn2
  "Bus 1 "/RConn1 -- Three-Phase Series RLC Branch2/LConn1 -- Three-Phase Series RLC Branch7/LConn1
  Three-Phase Series RLC Load1/LConn3 -- Subsystem2/LConn2 -- "Bus 4 "/LConn3
  "Bus 8 "/RConn3 -- Subsystem8/LConn2 -- Three-Phase Transformer (Two Windings)4/LConn3
  "Bus 8 "/RConn2 -- Subsystem8/LConn3 -- Three-Phase Transformer (Two Windings)4/LConn2
  Three-Phase Transformer (Two Windings)4/LConn1 -- Subsystem8/LConn1 -- "Bus 8 "/RConn1
  Three-Phase Series RLC Load5/LConn2 -- Subsystem4/LConn3 -- "Bus 9 "/RConn2
  Three-Phase Series RLC Load5/LConn3 -- Subsystem4/LConn1 -- "Bus 9 "/RConn3
  " Generator"/RConn2 -- Three-Phase Transformer (Two Windings)1/LConn2
  Three-Phase Series RLC Load1/LConn2 -- "Bus 4 "/LConn2 -- Subsystem2/LConn3
  Three-Phase Series RLC Load3/LConn1 -- Subsystem10/LConn1 -- "Bus 5 "/LConn1
  Three-Phase Series RLC Load3/LConn3 -- Subsystem10/LConn2 -- "Bus 5 "/LConn3
  "Bus 7 "/LConn3 -- Three-Phase Series RLC Branch11/LConn3 -- Subsystem11/LConn2
  Three-Phase Series RLC Load3/LConn2 -- Subsystem10/LConn3 -- "Bus 5 "/LConn2
  Three-Phase Series RLC Load10/LConn3 -- Three-Phase V-I Measurement3/LConn3 -- "Bus 14 "/RConn3
  Three-Phase Series RLC Load10/LConn2 -- Three-Phase V-I Measurement3/LConn2 -- "Bus 14 "/RConn2
  Three-Phase Series RLC Load10/LConn1 -- Three-Phase V-I Measurement3/LConn1 -- "Bus 14 "/RConn1
  Three-Phase Series RLC Load9/LConn3 -- Subsystem3/LConn2 -- "Bus 13 "/RConn3
  Three-Phase Series RLC Load9/LConn2 -- Subsystem3/LConn3 -- "Bus 13 "/RConn2
  Three-Phase Series RLC Load9/LConn1 -- "Bus 13 "/RConn1 -- Subsystem3/LConn1
  Three-Phase Series RLC Load8/LConn3 -- Subsystem5/LConn2 -- "Bus 12 "/RConn3
  Three-Phase Series RLC Load8/LConn2 -- Subsystem5/LConn3 -- "Bus 12 "/RConn2
  Three-Phase Series RLC Load8/LConn1 -- Subsystem5/LConn1 -- "Bus 12 "/RConn1
  Three-Phase Series RLC Load7/LConn3 -- Subsystem6/LConn2 -- "Bus 11 "/RConn3
  "Bus 11 "/RConn2 -- Subsystem6/LConn3 -- Three-Phase Series RLC Load7/LConn2
  "Bus 11 "/RConn1 -- Subsystem6/LConn1 -- Three-Phase Series RLC Load7/LConn1
  Three-Phase Series RLC Load6/LConn3 -- Subsystem7/LConn2 -- "Bus 10 "/RConn3
  Three-Phase Series RLC Load6/LConn2 -- Subsystem7/LConn3 -- "Bus 10 "/RConn2
  Three-Phase Series RLC Load6/LConn1 -- Subsystem7/LConn1 -- "Bus 10 "/RConn1
  Three-Phase Series RLC Load11/LConn3 -- Three-Phase Transformer (Two Windings)1/RConn3 -- "Bus 2 "/LConn3 -- Subsystem/LConn2
  Three-Phase Series RLC Branch9/LConn1 -- "Bus 8 "/LConn1
  Three-Phase Series RLC Branch9/LConn2 -- "Bus 8 "/LConn2
  Three-Phase Series RLC Branch9/LConn3 -- "Bus 8 "/LConn3
  Three-Phase Series RLC Load1/LConn1 -- Subsystem2/LConn1 -- "Bus 4 "/LConn1
  Three-Phase Series RLC Branch11/LConn2 -- Subsystem11/LConn3 -- "Bus 7 "/LConn2
  Three-Phase Series RLC Branch11/LConn1 -- Subsystem11/LConn1 -- "Bus 7 "/LConn1
  Three-Phase Transformer (Two Windings)5/RConn2 -- Subsystem1/LConn2 -- "Bus 1 "/LConn2
  Three-Phase Transformer (Two Windings)5/RConn1 -- Subsystem1/LConn3 -- "Bus 1 "/LConn1
  " Generator1"/RConn2 -- Three-Phase Transformer (Two Windings)5/LConn2
  Three-Phase Transformer (Two Windings)5/RConn3 -- Subsystem1/LConn1 -- "Bus 1 "/LConn3
  Three-Phase Transformer (Two Windings)2/RConn2 -- "Bus 3 "/LConn2 -- Subsystem9/LConn3 -- Three-Phase Series RLC Load12/LConn2
  Three-Phase Transformer (Two Windings)2/RConn1 -- "Bus 3 "/LConn1 -- Subsystem9/LConn1 -- Three-Phase Series RLC Load12/LConn1
  Synchronous Compensator/RConn2 -- Three-Phase Transformer (Two Windings)2/LConn2
  Three-Phase Transformer (Two Windings)2/RConn3 -- "Bus 3 "/LConn3 -- Subsystem9/LConn2 -- Three-Phase Series RLC Load12/LConn3
  "Bus 6 "/LConn2 -- Three-Phase Transformer (Two Windings)3/RConn2 -- Three-Phase V-I Measurement/LConn2 -- Three-Phase Series RLC Load4/LConn2
  "Bus 6 "/LConn1 -- Three-Phase Transformer (Two Windings)3/RConn1 -- Three-Phase V-I Measurement/LConn1 -- Three-Phase Series RLC Load4/LConn1
  Three-Phase Transformer (Two Windings)3/RConn3 -- "Bus 6 "/LConn3 -- Three-Phase Series RLC Load4/LConn3 -- Three-Phase V-I Measurement/LConn3
  "Synchronous Compensator "/RConn2 -- Three-Phase Transformer (Two Windings)3/LConn2
  "Bus 4 "/RConn3 -- Three-Phase Series RLC Branch1/LConn3 -- Three-Phase Series RLC Branch5/RConn3 -- Three-Phase Series RLC Branch6/RConn3 -- Three-Phase Series RLC Branch10/LConn3 -- Three-Phase Series RLC Branch8/RConn3
  "Bus 4 "/RConn2 -- Three-Phase Series RLC Branch1/LConn2 -- Three-Phase Series RLC Branch5/RConn2 -- Three-Phase Series RLC Branch6/RConn2 -- Three-Phase Series RLC Branch10/LConn2 -- Three-Phase Series RLC Branch8/RConn2
  "Bus 4 "/RConn1 -- Three-Phase Series RLC Branch1/LConn1 -- Three-Phase Series RLC Branch6/RConn1 -- Three-Phase Series RLC Branch10/LConn1 -- Three-Phase Series RLC Branch8/RConn1 -- Three-Phase Series RLC Branch5/RConn1
  Synchronous Compensator/RConn2 -- Three-Phase Transformer (Two Windings)4/RConn2
  Synchronous Compensator/RConn3 -- Three-Phase Transformer (Two Windings)4/RConn3
  Synchronous Compensator/RConn1 -- Three-Phase Transformer (Two Windings)4/RConn1
  "Synchronous Compensator "/RConn1 -- Three-Phase Transformer (Two Windings)3/LConn1
  "Synchronous Compensator "/RConn3 -- Three-Phase Transformer (Two Windings)3/LConn3
  " Generator1"/RConn3 -- Three-Phase Transformer (Two Windings)5/LConn3
  " Generator1"/RConn1 -- Three-Phase Transformer (Two Windings)5/LConn1
  Synchronous Compensator/RConn3 -- Three-Phase Transformer (Two Windings)2/LConn3
  Synchronous Compensator/RConn1 -- Three-Phase Transformer (Two Windings)2/LConn1
  " Generator"/RConn1 -- Three-Phase Transformer (Two Windings)1/LConn1
  " Generator"/RConn3 -- Three-Phase Transformer (Two Windings)1/LConn3
  "Bus 3 "/RConn3 -- Three-Phase Series RLC Branch5/LConn3 -- Three-Phase Series RLC Branch3/RConn3
  Three-Phase Transformer (Two Windings)1/RConn2 -- Three-Phase Series RLC Load11/LConn2 -- "Bus 2 "/LConn2 -- Subsystem/LConn3
  Three-Phase Series RLC Load5/LConn1 -- Subsystem4/LConn2 -- "Bus 9 "/RConn1

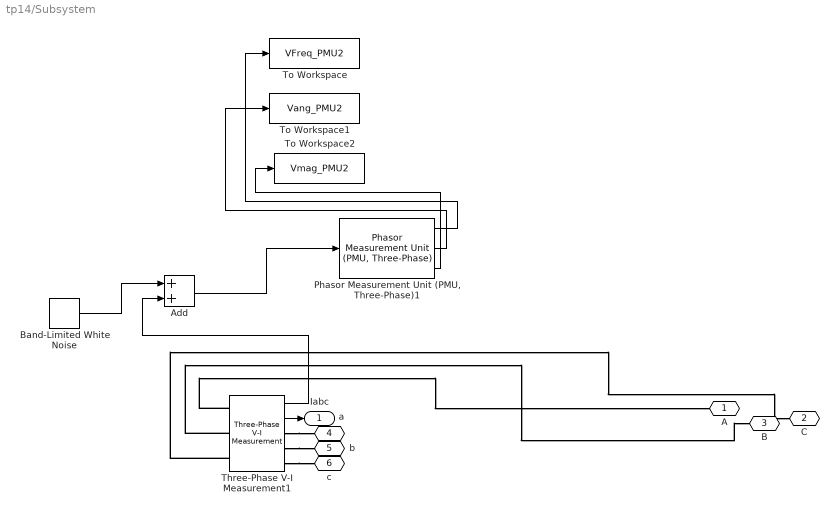
== system tp14/Subsystem ==
  Add : Sum
  Band-Limited White Noise : simulink/Sources/Band-Limited White Noise  Cov=3.16e-8  Ts=0.00833  seed=[23341]
  "Phasor Measurement Unit (PMU, Three-Phase)1" : eePMU/Phasor Measurement Unit (PMU, Three-Phase)  frequency=60  Nsr=64  k=2
      settings: LibrarySourceBlock=|
      | ee_sl_lib/Measurements/Phasor Measurement Unit
      | (PMU, Three-Phase)
  Three-Phase V-I Measurement1 : spsThreePhaseVIMeasurementLib/Three-Phase V-I Measurement  VoltageMeasurement=phase-to-ground  SetLabelV=off  LabelV=Vabc  Vpu=off  VpuLL=off  CurrentMeasurement=yes  SetLabelI=off  LabelI=Iabc  Ipu=off  Pbase=100e6  Vbase=500e3  OutputType=Complex  PhasorSimulation=off  PSBequivalent=0
  To Workspace : ToWorkspace  VariableName=VFreq_PMU2  SaveFormat=Timeseries  SampleTime=-1
  To Workspace1 : ToWorkspace  VariableName=Vang_PMU2  SaveFormat=Timeseries  SampleTime=-1
  To Workspace2 : ToWorkspace  VariableName=Vmag_PMU2  SaveFormat=Timeseries  SampleTime=-1
  A : PMIOPort  Side=Left
  C : PMIOPort  Port=2  Side=Left
  B : PMIOPort  Port=3  Side=Left
  a : PMIOPort  Port=4  Side=Right
  b : PMIOPort  Port=5  Side=Right
  c : PMIOPort  Port=6  Side=Right
  Iabc : Outport
  wires:
  Band-Limited White Noise/1 -> Add/1
  "Phasor Measurement Unit (PMU, Three-Phase)1"/2 -> To Workspace1/1
  Three-Phase V-I Measurement1/2 -> Iabc/1
  Add/1 -> "Phasor Measurement Unit (PMU, Three-Phase)1"/1
  "Phasor Measurement Unit (PMU, Three-Phase)1"/1 -> To Workspace/1
  Three-Phase V-I Measurement1/1 -> Add/2
  "Phasor Measurement Unit (PMU, Three-Phase)1"/3 -> To Workspace2/1
  connections:
  Three-Phase V-I Measurement1/LConn2 -- B/RConn1
  Three-Phase V-I Measurement1/RConn3 -- c/RConn1
  Three-Phase V-I Measurement1/RConn1 -- a/RConn1
  Three-Phase V-I Measurement1/RConn2 -- b/RConn1
  Three-Phase V-I Measurement1/LConn3 -- C/RConn1
  Three-Phase V-I Measurement1/LConn1 -- A/RConn1

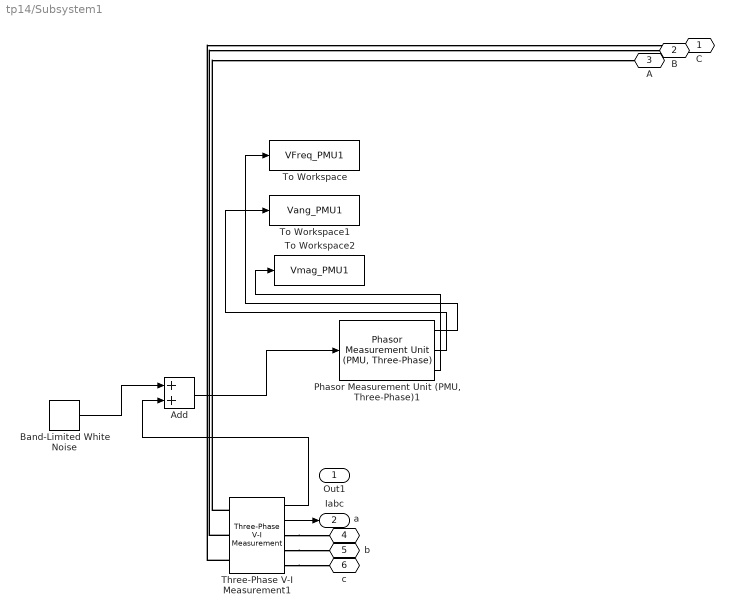
== system tp14/Subsystem1 ==
  Add : Sum
  Band-Limited White Noise : simulink/Sources/Band-Limited White Noise  Cov=3.16e-8  Ts=0.00833  seed=[23341]
  "Phasor Measurement Unit (PMU, Three-Phase)1" : eePMU/Phasor Measurement Unit (PMU, Three-Phase)  frequency=60  Nsr=64  k=2
  Three-Phase V-I Measurement1 : spsThreePhaseVIMeasurementLib/Three-Phase V-I Measurement  VoltageMeasurement=phase-to-ground  SetLabelV=off  LabelV=Vabc  Vpu=off  VpuLL=off  CurrentMeasurement=yes  SetLabelI=off  LabelI=Iabc  Ipu=off  Pbase=100e6  Vbase=500e3  OutputType=Complex  PhasorSimulation=off  PSBequivalent=0
  To Workspace : ToWorkspace  VariableName=VFreq_PMU1  SaveFormat=Timeseries  SampleTime=-1
  To Workspace1 : ToWorkspace  VariableName=Vang_PMU1  SaveFormat=Timeseries  SampleTime=-1
  To Workspace2 : ToWorkspace  VariableName=Vmag_PMU1  SaveFormat=Timeseries  SampleTime=-1
  C : PMIOPort  Side=Left
  B : PMIOPort  Port=2  Side=Left
  A : PMIOPort  Port=3  Side=Left
  a : PMIOPort  Port=4  Side=Right
  b : PMIOPort  Port=5  Side=Right
  c : PMIOPort  Port=6  Side=Right
  Out1 : Outport
  Iabc : Outport  Port=2
  wires:
  Band-Limited White Noise/1 -> Add/1
  "Phasor Measurement Unit (PMU, Three-Phase)1"/2 -> To Workspace1/1
  Add/1 -> "Phasor Measurement Unit (PMU, Three-Phase)1"/1
  "Phasor Measurement Unit (PMU, Three-Phase)1"/1 -> To Workspace/1
  "Phasor Measurement Unit (PMU, Three-Phase)1"/3 -> To Workspace2/1
  Three-Phase V-I Measurement1/1 -> Add/2
  Three-Phase V-I Measurement1/2 -> Iabc/1
  connections:
  Three-Phase V-I Measurement1/LConn3 -- C/RConn1
  Three-Phase V-I Measurement1/LConn2 -- B/RConn1
  Three-Phase V-I Measurement1/RConn2 -- b/RConn1
  Three-Phase V-I Measurement1/LConn1 -- A/RConn1
  Three-Phase V-I Measurement1/RConn1 -- a/RConn1
  Three-Phase V-I Measurement1/RConn3 -- c/RConn1

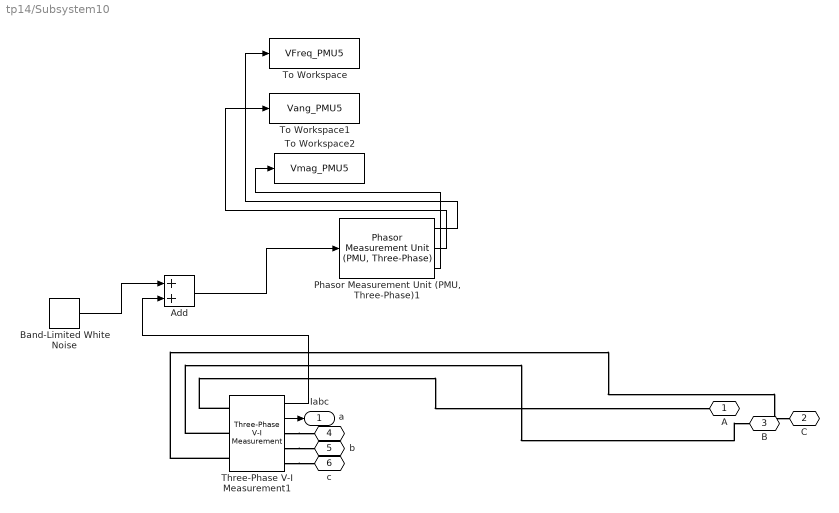
== system tp14/Subsystem10 ==
  Add : Sum
  Band-Limited White Noise : simulink/Sources/Band-Limited White Noise  Cov=3.16e-8  Ts=0.00833  seed=[23341]
  "Phasor Measurement Unit (PMU, Three-Phase)1" : eePMU/Phasor Measurement Unit (PMU, Three-Phase)  frequency=60  Nsr=64  k=2
  Three-Phase V-I Measurement1 : spsThreePhaseVIMeasurementLib/Three-Phase V-I Measurement  VoltageMeasurement=phase-to-ground  SetLabelV=off  LabelV=Vabc  Vpu=off  VpuLL=off  CurrentMeasurement=yes  SetLabelI=off  LabelI=Iabc  Ipu=off  Pbase=100e6  Vbase=500e3  OutputType=Complex  PhasorSimulation=off  PSBequivalent=0
  To Workspace : ToWorkspace  VariableName=VFreq_PMU5  SaveFormat=Timeseries  SampleTime=-1
  To Workspace1 : ToWorkspace  VariableName=Vang_PMU5  SaveFormat=Timeseries  SampleTime=-1
  To Workspace2 : ToWorkspace  VariableName=Vmag_PMU5  SaveFormat=Timeseries  SampleTime=-1
  A : PMIOPort  Side=Left
  C : PMIOPort  Port=2  Side=Left
  B : PMIOPort  Port=3  Side=Left
  a : PMIOPort  Port=4  Side=Right
  b : PMIOPort  Port=5  Side=Right
  c : PMIOPort  Port=6  Side=Right
  Iabc : Outport
  wires:
  Band-Limited White Noise/1 -> Add/1
  "Phasor Measurement Unit (PMU, Three-Phase)1"/2 -> To Workspace1/1
  Three-Phase V-I Measurement1/2 -> Iabc/1
  Add/1 -> "Phasor Measurement Unit (PMU, Three-Phase)1"/1
  "Phasor Measurement Unit (PMU, Three-Phase)1"/1 -> To Workspace/1
  Three-Phase V-I Measurement1/1 -> Add/2
  "Phasor Measurement Unit (PMU, Three-Phase)1"/3 -> To Workspace2/1
  connections:
  Three-Phase V-I Measurement1/LConn2 -- B/RConn1
  Three-Phase V-I Measurement1/RConn3 -- c/RConn1
  Three-Phase V-I Measurement1/RConn1 -- a/RConn1
  Three-Phase V-I Measurement1/RConn2 -- b/RConn1
  Three-Phase V-I Measurement1/LConn3 -- C/RConn1
  Three-Phase V-I Measurement1/LConn1 -- A/RConn1

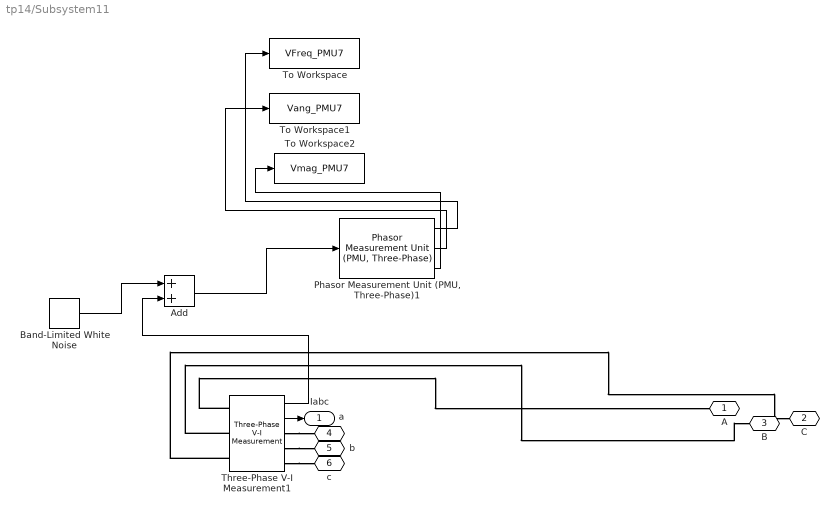
== system tp14/Subsystem11 ==
  Add : Sum
  Band-Limited White Noise : simulink/Sources/Band-Limited White Noise  Cov=3.16e-8  Ts=0.00833  seed=[23341]
  "Phasor Measurement Unit (PMU, Three-Phase)1" : eePMU/Phasor Measurement Unit (PMU, Three-Phase)  frequency=60  Nsr=64  k=2
  Three-Phase V-I Measurement1 : spsThreePhaseVIMeasurementLib/Three-Phase V-I Measurement  VoltageMeasurement=phase-to-ground  SetLabelV=off  LabelV=Vabc  Vpu=off  VpuLL=off  CurrentMeasurement=yes  SetLabelI=off  LabelI=Iabc  Ipu=off  Pbase=100e6  Vbase=500e3  OutputType=Complex  PhasorSimulation=off  PSBequivalent=0
  To Workspace : ToWorkspace  VariableName=VFreq_PMU7  SaveFormat=Timeseries  SampleTime=-1
  To Workspace1 : ToWorkspace  VariableName=Vang_PMU7  SaveFormat=Timeseries  SampleTime=-1
  To Workspace2 : ToWorkspace  VariableName=Vmag_PMU7  SaveFormat=Timeseries  SampleTime=-1
  A : PMIOPort  Side=Left
  C : PMIOPort  Port=2  Side=Left
  B : PMIOPort  Port=3  Side=Left
  a : PMIOPort  Port=4  Side=Right
  b : PMIOPort  Port=5  Side=Right
  c : PMIOPort  Port=6  Side=Right
  Iabc : Outport
  wires:
  Band-Limited White Noise/1 -> Add/1
  "Phasor Measurement Unit (PMU, Three-Phase)1"/2 -> To Workspace1/1
  Three-Phase V-I Measurement1/2 -> Iabc/1
  Add/1 -> "Phasor Measurement Unit (PMU, Three-Phase)1"/1
  "Phasor Measurement Unit (PMU, Three-Phase)1"/1 -> To Workspace/1
  Three-Phase V-I Measurement1/1 -> Add/2
  "Phasor Measurement Unit (PMU, Three-Phase)1"/3 -> To Workspace2/1
  connections:
  Three-Phase V-I Measurement1/LConn2 -- B/RConn1
  Three-Phase V-I Measurement1/RConn3 -- c/RConn1
  Three-Phase V-I Measurement1/RConn1 -- a/RConn1
  Three-Phase V-I Measurement1/RConn2 -- b/RConn1
  Three-Phase V-I Measurement1/LConn3 -- C/RConn1
  Three-Phase V-I Measurement1/LConn1 -- A/RConn1

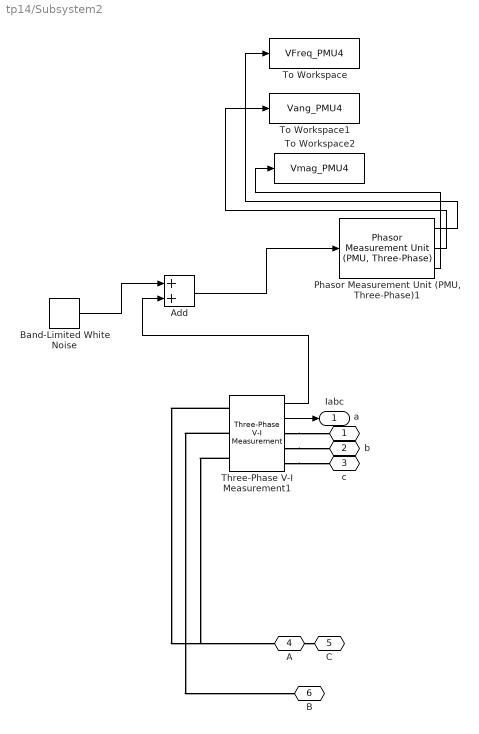
== system tp14/Subsystem2 ==
  Add : Sum
  Band-Limited White Noise : simulink/Sources/Band-Limited White Noise  Cov=3.16e-8  Ts=0.00833  seed=[23341]
  "Phasor Measurement Unit (PMU, Three-Phase)1" : eePMU/Phasor Measurement Unit (PMU, Three-Phase)  frequency=60  Nsr=64  k=2
  Three-Phase V-I Measurement1 : spsThreePhaseVIMeasurementLib/Three-Phase V-I Measurement  VoltageMeasurement=phase-to-ground  SetLabelV=off  LabelV=Vabc  Vpu=off  VpuLL=off  CurrentMeasurement=yes  SetLabelI=off  LabelI=Iabc  Ipu=off  Pbase=100e6  Vbase=500e3  OutputType=Complex  PhasorSimulation=off  PSBequivalent=0
  To Workspace : ToWorkspace  VariableName=VFreq_PMU4  SaveFormat=Timeseries  SampleTime=-1
  To Workspace1 : ToWorkspace  VariableName=Vang_PMU4  SaveFormat=Timeseries  SampleTime=-1
  To Workspace2 : ToWorkspace  VariableName=Vmag_PMU4  SaveFormat=Timeseries  SampleTime=-1
  a : PMIOPort  Side=Right
  b : PMIOPort  Port=2  Side=Right
  c : PMIOPort  Port=3  Side=Right
  A : PMIOPort  Port=4  Side=Left
  C : PMIOPort  Port=5  Side=Left
  B : PMIOPort  Port=6  Side=Left
  Iabc : Outport
  wires:
  "Phasor Measurement Unit (PMU, Three-Phase)1"/3 -> To Workspace2/1
  "Phasor Measurement Unit (PMU, Three-Phase)1"/1 -> To Workspace/1
  Add/1 -> "Phasor Measurement Unit (PMU, Three-Phase)1"/1
  Three-Phase V-I Measurement1/1 -> Add/2
  "Phasor Measurement Unit (PMU, Three-Phase)1"/2 -> To Workspace1/1
  Band-Limited White Noise/1 -> Add/1
  Three-Phase V-I Measurement1/2 -> Iabc/1
  connections:
  Three-Phase V-I Measurement1/LConn2 -- B/RConn1
  Three-Phase V-I Measurement1/RConn2 -- b/RConn1
  Three-Phase V-I Measurement1/LConn3 -- C/RConn1
  Three-Phase V-I Measurement1/RConn1 -- a/RConn1
  Three-Phase V-I Measurement1/RConn3 -- c/RConn1
  Three-Phase V-I Measurement1/LConn1 -- A/RConn1

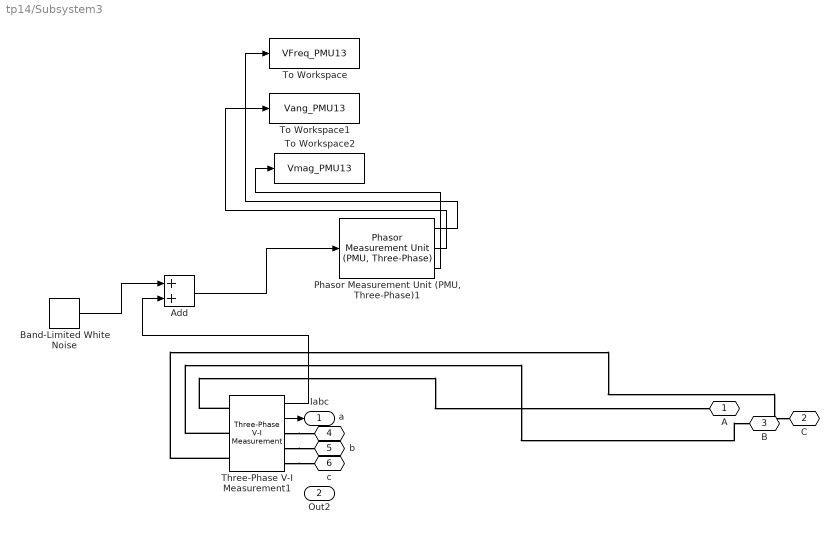
== system tp14/Subsystem3 ==
  Add : Sum
  Band-Limited White Noise : simulink/Sources/Band-Limited White Noise  Cov=3.16e-8  Ts=0.00833  seed=[23341]
  "Phasor Measurement Unit (PMU, Three-Phase)1" : eePMU/Phasor Measurement Unit (PMU, Three-Phase)  frequency=60  Nsr=64  k=2
  Three-Phase V-I Measurement1 : spsThreePhaseVIMeasurementLib/Three-Phase V-I Measurement  VoltageMeasurement=phase-to-ground  SetLabelV=off  LabelV=Vabc  Vpu=off  VpuLL=off  CurrentMeasurement=yes  SetLabelI=off  LabelI=Iabc  Ipu=off  Pbase=100e6  Vbase=500e3  OutputType=Complex  PhasorSimulation=off  PSBequivalent=0
  To Workspace : ToWorkspace  VariableName=VFreq_PMU13  SaveFormat=Timeseries  SampleTime=-1
  To Workspace1 : ToWorkspace  VariableName=Vang_PMU13  SaveFormat=Timeseries  SampleTime=-1
  To Workspace2 : ToWorkspace  VariableName=Vmag_PMU13  SaveFormat=Timeseries  SampleTime=-1
  A : PMIOPort  Side=Left
  C : PMIOPort  Port=2  Side=Left
  B : PMIOPort  Port=3  Side=Left
  a : PMIOPort  Port=4  Side=Right
  b : PMIOPort  Port=5  Side=Right
  c : PMIOPort  Port=6  Side=Right
  Iabc : Outport
  Out2 : Outport  Port=2
  wires:
  Band-Limited White Noise/1 -> Add/1
  "Phasor Measurement Unit (PMU, Three-Phase)1"/2 -> To Workspace1/1
  Three-Phase V-I Measurement1/2 -> Iabc/1
  Add/1 -> "Phasor Measurement Unit (PMU, Three-Phase)1"/1
  "Phasor Measurement Unit (PMU, Three-Phase)1"/1 -> To Workspace/1
  Three-Phase V-I Measurement1/1 -> Add/2
  "Phasor Measurement Unit (PMU, Three-Phase)1"/3 -> To Workspace2/1
  connections:
  Three-Phase V-I Measurement1/LConn2 -- B/RConn1
  Three-Phase V-I Measurement1/RConn3 -- c/RConn1
  Three-Phase V-I Measurement1/RConn1 -- a/RConn1
  Three-Phase V-I Measurement1/RConn2 -- b/RConn1
  Three-Phase V-I Measurement1/LConn3 -- C/RConn1
  Three-Phase V-I Measurement1/LConn1 -- A/RConn1
